simulink model "furuta2"  (R2022b)
settings: Solver=VariableStepAuto  StartTime=0.0  StopTime=10  FixedStep=1  MaxStep=0.09  MinStep=0.00001  RelTol=1e-10  AbsTol=2
values from neighbouring files (symbols this model uses):
  c1 = 0.005    [mathlab_modeling.m]
  c2 = 0.5    [mathlab_modeling.m]
  J = 0.0023    [mathlab_modeling.m]
  J2 = 1/3 * m2 * l2^2    (= 2.45e-05)    [mathlab_modeling.m]
  ke = 0.395    [mathlab_modeling.m]
  km = 0.395    [mathlab_modeling.m]
  L = 0.087    [mathlab_modeling.m]
  l1 = 0.1    [mathlab_modeling.m]
  l2 = 0.07    [mathlab_modeling.m]
  m2 = 0.015    [mathlab_modeling.m]
  Mtr = 0.01    [mathlab_modeling.m]
  R = 5.485    [mathlab_modeling.m]
  start = (90 - start) * pi / 180    (= 1.65806278939)    [mathlab_modeling.m]
  tm = 0.01    [mathlab_modeling.m]
libraries: slpidlib x1
settings Model: Creator=Дарья  LastModifiedBy=Дарья

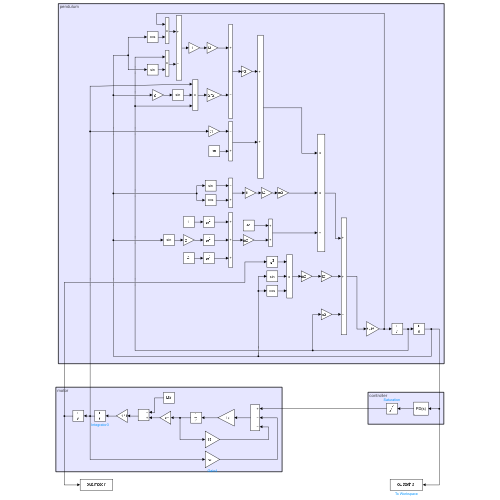
[thumbnail: Simulink's stored preview of the top-level diagram]
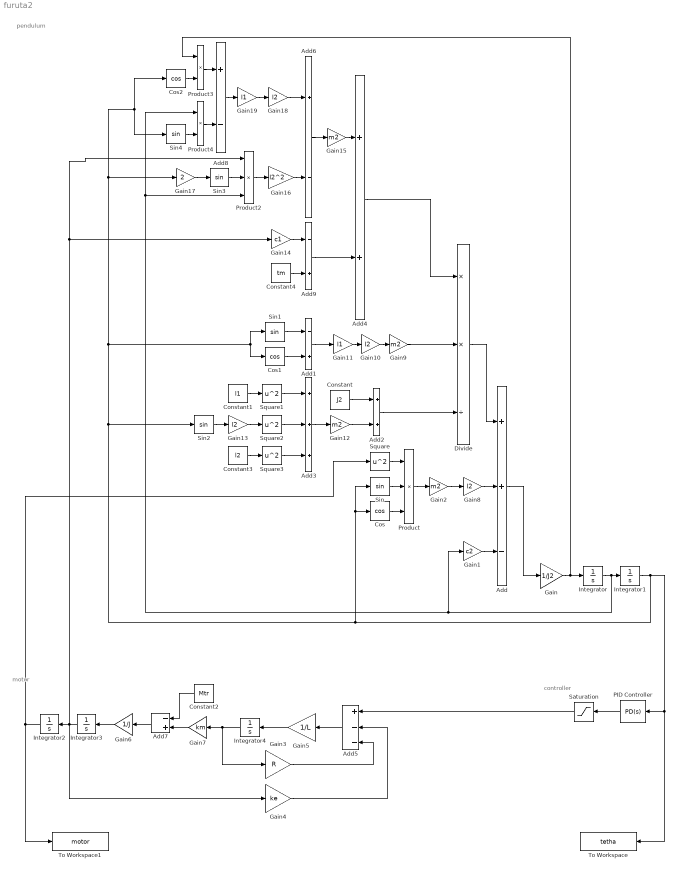
== system furuta2 ==
  note: motor
  note: controller
  note: pendulum
  Add : Sum  Inputs=++-
  Add1 : Sum  Inputs=-+
  Add2 : Sum
  Add3 : Sum  Inputs=+++
  Add4 : Sum
  Add5 : Sum  Inputs=+--
  Add6 : Sum  Inputs=+-
  Add7 : Sum  Inputs=-+
  Add8 : Sum  Inputs=+-
  Add9 : Sum  Inputs=-+
  Constant : Constant  Value=J2
  Constant1 : Constant  Value=l1
  Constant2 : Constant  Value=Mtr
  Constant3 : Constant  Value=l2
  Constant4 : Constant  Value=tm
  Cos : Trigonometry  Operator=cos
  Cos1 : Trigonometry  Operator=cos
  Cos2 : Trigonometry  Operator=cos
  Divide : Product  Inputs=**/
  Gain : Gain  Gain=1/J2
  Gain1 : Gain  Gain=c2
  Gain{8,10,13,18} (4 alike) : Gain  Gain=l2
  Gain11 : Gain  Gain=l1
  Gain{2,9,12,15} (4 alike) : Gain  Gain=m2
  Gain14 : Gain  Gain=c1
  Gain16 : Gain  Gain=l2^2
  Gain17 : Gain  Gain=2
  Gain19 : Gain  Gain=l1
  Gain3 : Gain  Gain=R
  Gain4 : Gain  Gain=ke
  Gain5 : Gain  Gain=1/L
  Gain6 : Gain  Gain=1/J
  Gain7 : Gain  Gain=km
  Integrator{,2..4} (4 alike) : Integrator
  Integrator1 : Integrator  InitialCondition=start
  PID Controller : slpidlib/PID Controller  Controller=PD  Form=Parallel  TimeDomain=Continuous-time  UseExternalTs=off  SampleTime=-1  IntegratorMethod=Forward Euler  FilterMethod=Forward Euler  ControllerParametersSource=internal  P=13.5  I=0  UseKiTs=off  D=10  N=100  UseFilter=on  TunerSelectOption=Transfer Function Based (PID Tuner App)  InitialConditionSource=internal  InitialConditionForIntegrator=0  InitialConditionForFilter=0  DifferentiatorICPrevScaledInput=0  ExternalReset=none  TrackingMode=off  Kt=1  LimitOutput=off  SatLimitsSource=internal  UpperSaturationLimit=inf  LowerSaturationLimit=-inf  LinearizeAsGain=on  AntiWindupMode=none  Kb=1  LimitIntegrator=off  UpperIntegratorSaturationLimit=inf  LowerIntegratorSaturationLimit=-inf  POutMin=[]  POutMax=[]  IOutMin=[]  IOutMax=[]  DOutMin=[]  DOutMax=[]  NOutMin=[]  NOutMax=[]  SumOutMin=[]  SumOutMax=[]  SaturationOutMin=[]  SaturationOutMax=[]  PParamMin=[]  PParamMax=[]  IParamMin=[]  IParamMax=[]  DParamMin=[]  DParamMax=[]  NParamMin=[]  NParamMax=[]  KbParamMin=[]  KbParamMax=[]  KtParamMin=[]  KtParamMax=[]  KbOutMin=[]  KbOutMax=[]  KtOutMin=[]  KtOutMax=[]  IntegratorOutMin=[]  IntegratorOutMax=[]  FilterOutMin=[]  FilterOutMax=[]  SumI1OutMin=[]  SumI1OutMax=[]  SumI2OutMin=[]  SumI2OutMax=[]  SumI3OutMin=[]  SumI3OutMax=[]  SumI4OutMin=[]  SumI4OutMax=[]  SumDOutMin=[]  SumDOutMax=[]  DifferentiatorOutMin=[]  DifferentiatorOutMax=[]  FilterDiffOutCoefMin=[]  FilterDiffOutCoefMax=[]  ReciprocalOutMin=[]  ReciprocalOutMax=[]  SumDenOutMin=[]  SumDenOutMax=[]  SumNumOutMin=[]  SumNumOutMax=[]  DivideOutMin=[]  DivideOutMax=[]  UdiffTsProdOutMin=[]  UdiffTsProdOutMax=[]  NTsProdOutMin=[]  NTsProdOutMax=[]  UintegralTsProdOutMin=[]  UintegralTsProdOutMax=[]  UngainTsProdOutMin=[]  UngainTsProdOutMax=[]  ClampingZeroOutDataTypeStr=Inherit: Inherit via back propagation  ClampingZeroOutMin=[]  ClampingZeroOutMax=[]  FilterDenConstantOutDataTypeStr=Inherit: Inherit via back propagation  FilterDenConstantOutMin=[]  FilterDenConstantOutMax=[]  PCopyOutDataTypeStr=Inherit: Inherit via back propagation  PCopyOutMin=[]  PCopyOutMax=[]  NCopyOutDataTypeStr=Inherit: Inherit via back propagation  NCopyOutMin=[]  NCopyOutMax=[]  IntegratorContinuousStateAttributes=''  IntegratorStateMustResolveToSignalObject=off  IntegratorRTWStateStorageClass=Auto  FilterContinuousStateAttributes=''  FilterStateMustResolveToSignalObject=off  FilterRTWStateStorageClass=Auto  ParallelPVariant=InternalParameters  IdealPVariant=Disabled  IVariant=Disabled  DVariant=InternalParameters  IntegratorVariant=Disabled  SatVariant=Disabled  AWVariant=Disabled  PCopyVariant=Disabled  TRVariant=Disabled  FdbkBlocksVariant=Forward  IdealPFdbkVariant=Disabled  SatFdbkVariant=Disabled  DerivativeFilterVariant=ContFilter  NVariant=InternalParameters  NCopyVariant=Disabled  FilterICVariant=InternalICsFilter  IntegratorICVariant=Disabled  ExternalResetVariant=Disabled  TRSumVariant=Passthrough  SumFdbkVariant=Disabled  SumVariant=Sum_PD  TsampFilterVariant=InternalTs  TsampNgainVariant=Passthrough  TsampIntegralVariant=Disabled_SignalSpec  ExternalSaturationOutDataTypeStr=Inherit: Same as second input
  Product : Product  Inputs=3
  Product2 : Product  Inputs=3
  Product3 : Product
  Product4 : Product
  Saturation : Saturate  UpperLimit=2500  LowerLimit=-2500
  Sin{,1..4} (5 alike) : Trigonometry
  Square{,1..3} (4 alike) : Math  Operator=square
  To Workspace : ToWorkspace  VariableName=tetha  SaveFormat=Timeseries  SampleTime=-1
  To Workspace1 : ToWorkspace  VariableName=motor  SaveFormat=Timeseries  SampleTime=-1
  wires:
  Integrator/1 -> Product4/1, Product2/3, Gain1/1, Integrator1/1
  Gain7/1 -> Add7/2
  Gain3/1 -> Add5/3
  Add5/1 -> Gain5/1
  Gain6/1 -> Integrator3/1
  Constant2/1 -> Add7/1
  Gain5/1 -> Integrator4/1
  Gain4/1 -> Add5/2
  Integrator4/1 -> Gain3/1, Gain7/1
  Add7/1 -> Gain6/1
  PID Controller/1 -> Saturation/1
  Add/1 -> Gain/1
  Gain1/1 -> Add/3
  Gain2/1 -> Gain8/1
  Gain8/1 -> Add/2
  Product/1 -> Gain2/1
  Cos/1 -> Product/3
  Sin/1 -> Product/2
  Square/1 -> Product/1
  Integrator2/1 -> To Workspace1/1, Square/1
  Gain9/1 -> Divide/2
  Gain11/1 -> Gain10/1
  Gain10/1 -> Gain9/1
  Add1/1 -> Gain11/1
  Sin1/1 -> Add1/1
  Cos1/1 -> Add1/2
  Add2/1 -> Divide/3
  Constant/1 -> Add2/1
  Gain12/1 -> Add2/2
  Add3/1 -> Gain12/1
  Constant1/1 -> Square1/1
  Square1/1 -> Add3/1
  Square2/1 -> Add3/2
  Gain13/1 -> Square2/1
  Sin2/1 -> Gain13/1
  Constant3/1 -> Square3/1
  Square3/1 -> Add3/3
  Integrator3/1 -> Gain4/1, Integrator2/1, Gain14/1, Product2/1
  Gain15/1 -> Add4/1
  Add6/1 -> Gain15/1
  Sin3/1 -> Product2/2
  Gain17/1 -> Sin3/1
  Integrator1/1 -> Gain17/1, Cos2/1, Sin4/1, Sin1/1, Cos1/1, Sin2/1, Sin/1, Cos/1, To Workspace/1, PID Controller/1
  Product2/1 -> Gain16/1
  Gain16/1 -> Add6/2
  Gain18/1 -> Add6/1
  Gain19/1 -> Gain18/1
  Add8/1 -> Gain19/1
  Product3/1 -> Add8/1
  Cos2/1 -> Product3/2
  Gain/1 -> Integrator/1, Product3/1
  Product4/1 -> Add8/2
  Sin4/1 -> Product4/2
  Add4/1 -> Divide/1
  Gain14/1 -> Add9/1
  Constant4/1 -> Add9/2
  Add9/1 -> Add4/2
  Divide/1 -> Add/1
  Saturation/1 -> Add5/1
